simulink model "pet_integration_architecture"  (R2024a)
settings: Solver=FixedStepDiscrete  StartTime=0.0  StopTime=10.0  RelTol=1e-3
undefined symbols (not defined in the file or in its folder): D1, P
undefined symbols (not defined in the file): orig
(part 2 of 3)

== system pet_integration_architecture/Remote Data Server/Local WSL Store ==
  Bus Element In2 : Inport  PortName=win2wsl
  bash Scripts : Subsystem
      settings: PortSchema="{\"entries\":[{\"content\":{\"headerSize\":26,\"margin\":15,\"minimumSpacing\":25,\"sides\":[{\"content\":{},\"type\":\"ConnectorPlacement.EquallySpacedRectSide\",\"uuid\":\"97c1e145-3d4b-49de-9739-71f2af5be190\"},{\"content\":{\"side\":\"RIGHT\"},\"type\":\"ConnectorPlacement.EquallySpacedRectSide\",\"uuid\":\"5a937baa-e46f-4764-8b00-75a1eb9e59b0\"},{\"content\":{\"side\":\"TOP\"},\"type\":\"ConnectorPlacement.EquallySpacedRectSide\",\"uuid\":\"83b91a39-9e34-441d-bccf-4f6b71aa9c87\"}]},\"type\":\"ConnectorPlacement.EquallySpacedConnector\",\"uuid\":\"3f7bec2f-99ca-4d64-b419-ed6b2efa51c2\"}],\"packageUris\":[\"http://schema.mathworks.com/mf0/Connector/R2020b\"],\"version\":\"1.0\"}"
  slurm Jobs : Subsystem
      settings: PortSchema="{\"entries\":[{\"content\":{\"headerSize\":26,\"margin\":15,\"minimumSpacing\":25,\"sides\":[{\"content\":{},\"type\":\"ConnectorPlacement.EquallySpacedRectSide\",\"uuid\":\"97c1e145-3d4b-49de-9739-71f2af5be190\"},{\"content\":{\"side\":\"RIGHT\"},\"type\":\"ConnectorPlacement.EquallySpacedRectSide\",\"uuid\":\"5a937baa-e46f-4764-8b00-75a1eb9e59b0\"},{\"content\":{\"side\":\"TOP\"},\"type\":\"ConnectorPlacement.EquallySpacedRectSide\",\"uuid\":\"83b91a39-9e34-441d-bccf-4f6b71aa9c87\"}]},\"type\":\"ConnectorPlacement.EquallySpacedConnector\",\"uuid\":\"3f7bec2f-99ca-4d64-b419-ed6b2efa51c2\"}],\"packageUris\":[\"http://schema.mathworks.com/mf0/Connector/R2020b\"],\"version\":\"1.0\"}"
  sshConnect : Subsystem
      settings: PortSchema="{\"entries\":[{\"content\":{\"headerSize\":26,\"margin\":15,\"minimumSpacing\":25,\"sides\":[{\"content\":{},\"type\":\"ConnectorPlacement.EquallySpacedRectSide\",\"uuid\":\"97c1e145-3d4b-49de-9739-71f2af5be190\"},{\"content\":{\"side\":\"RIGHT\"},\"type\":\"ConnectorPlacement.EquallySpacedRectSide\",\"uuid\":\"5a937baa-e46f-4764-8b00-75a1eb9e59b0\"},{\"content\":{\"side\":\"TOP\"},\"type\":\"ConnectorPlacement.EquallySpacedRectSide\",\"uuid\":\"83b91a39-9e34-441d-bccf-4f6b71aa9c87\"}]},\"type\":\"ConnectorPlacement.EquallySpacedConnector\",\"uuid\":\"3f7bec2f-99ca-4d64-b419-ed6b2efa51c2\"}],\"packageUris\":[\"http://schema.mathworks.com/mf0/Connector/R2020b\"],\"version\":\"1.0\"}"
  Bus Element Out2 : Outport  AllowServiceAccess=on  PortName=rsync
  Bus Element Out1 : Outport  Port=2  PortName=wsl2win

== system pet_integration_architecture/Remote Data Server/Loris ==

== system pet_integration_architecture/Remote Data Server/Remote Execution Module ==
  Bus Element In1 : Inport  AllowServiceAccess=on  PortName=SSHPort
  In Bus Element1 : Inport  Port=2  PortName=rsync

== system pet_integration_architecture/Remote Data Server/SSH Connection Module ==
  Bus Element In2 : Inport  AllowServiceAccess=on  PortName=rsync
  Bus Element In1 : Inport  Port=2  AllowServiceAccess=on  PortName=SSHPort

== system pet_integration_architecture/Remote Data Server/StormRemote GUI ==

== system pet_integration_architecture/Remote Data Server/WSL Inteface Module ==
  Bus Element In2 : Inport  PortName=wsl2win
  Bus Element In1 : Inport  Port=2  AllowServiceAccess=on  PortName=remote.config
  Bus Element Out1 : Outport  PortName=win2wsl

== system pet_integration_architecture/Remote Data Server/importBIDSDataset ==
  Bus Element In1 : Inport  AllowServiceAccess=on  PortName=local.raw
  Bus Element Out1 : Outport  AllowServiceAccess=on  PortName=Derivatives

== system pet_integration_architecture/brainstorm SQLite Server/Freesurfer Processing Server ==
  Bus Element In1 : Inport  AllowServiceAccess=on  PortName=remote.raw
  PETSurfer : Subsystem
      settings: PortSchema="{\"entries\":[{\"content\":{\"headerSize\":26,\"margin\":15,\"minimumSpacing\":25,\"sides\":[{\"content\":{},\"type\":\"ConnectorPlacement.EquallySpacedRectSide\",\"uuid\":\"d99db108-8c8a-4010-81b2-f142fbf318f5\"},{\"content\":{\"connectorIds\":[\"Out1\"],\"side\":\"RIGHT\"},\"type\":\"ConnectorPlacement.EquallySpacedRectSide\",\"uuid\":\"9190d96c-22e3-4cc9-a507-8f094dc67743\"},{\"content\":{\"side\":\"TOP\"},\"type\":\"ConnectorPlacement.EquallySpacedRectSide\",\"uuid\":\"08b46875-eac1-4edb-b2eb-5598dd517a75\"}]},\"type\":\"ConnectorPlacement.EquallySpacedConnector\",\"uuid\":\"c8d2d02b-cf5a-431f-8876-22d36c8a9b33\"}],\"packageUris\":[\"http://schema.mathworks.com/mf0/Connector/R2020b\"],\"version\":\"1.0\"}"
  recon all : Subsystem
      settings: PortSchema="{\"entries\":[{\"content\":{\"headerSize\":26,\"margin\":15,\"minimumSpacing\":25,\"sides\":[{\"content\":{\"connectorIds\":[\"In1\"]},\"type\":\"ConnectorPlacement.EquallySpacedRectSide\",\"uuid\":\"1ec5f43e-86ec-4420-9dd8-c30b843d5131\"},{\"content\":{\"connectorIds\":[\"Out1\"],\"side\":\"RIGHT\"},\"type\":\"ConnectorPlacement.EquallySpacedRectSide\",\"uuid\":\"372e8174-47dc-4989-909e-f78b7a521fdc\"},{\"content\":{\"side\":\"TOP\"},\"type\":\"ConnectorPlacement.EquallySpacedRectSide\",\"uuid\":\"cc67dfee-4023-44ab-9dd9-de9f078f7d77\"}]},\"type\":\"ConnectorPlacement.EquallySpacedConnector\",\"uuid\":\"fe3e41a6-8f67-44d2-abc6-74b481cf0464\"}],\"packageUris\":[\"http://schema.mathworks.com/mf0/Connector/R2020b\"],\"version\":\"1.0\"}"
  Bus Element Out1 : Outport  PortName=freesurfer derivatives

== system pet_integration_architecture/brainstorm SQLite Server/LORIS Data Ingestor ==

== system pet_integration_architecture/brainstorm SQLite Server/Remote Data Server ==
  Bus Element In1 : Inport  PortName=Derivatives
  " sourceData" : Subsystem
      settings: PortSchema="{\"entries\":[{\"content\":{\"headerSize\":26,\"margin\":15,\"minimumSpacing\":25,\"sides\":[{\"content\":{},\"type\":\"ConnectorPlacement.EquallySpacedRectSide\",\"uuid\":\"a3539b9a-22db-4da3-b271-35b287ced3a1\"},{\"content\":{\"connectorIds\":[\"Out1\"],\"side\":\"RIGHT\"},\"type\":\"ConnectorPlacement.EquallySpacedRectSide\",\"uuid\":\"72d9f298-5062-46d4-b3c5-f2fa85d7a7a6\"},{\"content\":{\"side\":\"TOP\"},\"type\":\"ConnectorPlacement.EquallySpacedRectSide\",\"uuid\":\"050469fd-3881-4b53-a813-94df038aa659\"}]},\"type\":\"ConnectorPlacement.EquallySpacedConnector\",\"uuid\":\"6db04dad-62f3-4987-a6a9-d236db4fe2a3\"}],\"packageUris\":[\"http://schema.mathworks.com/mf0/Connector/R2020b\"],\"version\":\"1.0\"}"
  Home : Subsystem
      settings: PortSchema="{\"entries\":[{\"content\":{\"headerSize\":26,\"margin\":15,\"minimumSpacing\":25,\"sides\":[{\"content\":{\"connectorIds\":[\"Out1\"]},\"type\":\"ConnectorPlacement.EquallySpacedRectSide\",\"uuid\":\"a3539b9a-22db-4da3-b271-35b287ced3a1\"},{\"content\":{\"side\":\"RIGHT\"},\"type\":\"ConnectorPlacement.EquallySpacedRectSide\",\"uuid\":\"72d9f298-5062-46d4-b3c5-f2fa85d7a7a6\"},{\"content\":{\"side\":\"TOP\"},\"type\":\"ConnectorPlacement.EquallySpacedRectSide\",\"uuid\":\"050469fd-3881-4b53-a813-94df038aa659\"}]},\"type\":\"ConnectorPlacement.EquallySpacedConnector\",\"uuid\":\"6db04dad-62f3-4987-a6a9-d236db4fe2a3\"}],\"packageUris\":[\"http://schema.mathworks.com/mf0/Connector/R2020b\"],\"version\":\"1.0\"}"
  derivativesData : Subsystem
      settings: PortSchema="{\"entries\":[{\"content\":{\"headerSize\":26,\"margin\":15,\"minimumSpacing\":25,\"sides\":[{\"content\":{},\"type\":\"ConnectorPlacement.EquallySpacedRectSide\",\"uuid\":\"a3539b9a-22db-4da3-b271-35b287ced3a1\"},{\"content\":{\"side\":\"RIGHT\"},\"type\":\"ConnectorPlacement.EquallySpacedRectSide\",\"uuid\":\"72d9f298-5062-46d4-b3c5-f2fa85d7a7a6\"},{\"content\":{\"side\":\"TOP\"},\"type\":\"ConnectorPlacement.EquallySpacedRectSide\",\"uuid\":\"050469fd-3881-4b53-a813-94df038aa659\"}]},\"type\":\"ConnectorPlacement.EquallySpacedConnector\",\"uuid\":\"6db04dad-62f3-4987-a6a9-d236db4fe2a3\"}],\"packageUris\":[\"http://schema.mathworks.com/mf0/Connector/R2020b\"],\"version\":\"1.0\"}"
  Bus Element Out4 : Outport  AllowServiceAccess=on  PortName=sourceCode  Element=github
  Bus Element Out3 : Outport  Port=2  AllowServiceAccess=on  PortName=SSHPort
  Bus Element Out1 : Outport  Port=3  AllowServiceAccess=on  PortName=remote.raw
  Bus Element Out2 : Outport  Port=4  AllowServiceAccess=on  PortName=remote.derivatives
  wires:
  " sourceData"/1(remote) -> Bus Element Out1/1, Bus Element Out2/1
  Home/1(sourceCode) -> Bus Element Out4/1

== system pet_integration_architecture/brainstorm SQLite Server/create Virtual Environment ==

== system pet_integration_architecture/brainstorm SQLite Server/gitClone Brainstorm ==
  Bus Element In1 : Inport  AllowServiceAccess=on  PortName=sourceCode

== system pet_integration_architecture/brainstorm SQLite Server/jobScheduler ==

== system pet_integration_architecture/brainstorm SQLite Server/loadPython ==

== system pet_integration_architecture/brainstorm SQLite Server/processingSoftware ==

== system pet_integration_architecture/brainstorm core/bst_get ==

== system pet_integration_architecture/brainstorm core/bst_set ==

== system pet_integration_architecture/brainstorm database/Brainstorm Home Dir ==

== system pet_integration_architecture/brainstorm database/Brainstorm User Data  ==

== system pet_integration_architecture/brainstorm database/Brainstorm data server ==
  note: data directory
  note: anat directory
  note: /anat/subName/subject/
  note: /data/subName/@raw/
  Bus Element In1 : Inport  PortName=@db
  channel_ : Subsystem
      settings: PortSchema="{\"entries\":[{\"content\":{\"headerSize\":26,\"margin\":15,\"minimumSpacing\":25,\"sides\":[{\"content\":{\"connectorIds\":[\"In1\"]},\"type\":\"ConnectorPlacement.EquallySpacedRectSide\",\"uuid\":\"e452b68a-48a0-46a4-9e6b-6a7ab63d76ba\"},{\"content\":{\"side\":\"RIGHT\"},\"type\":\"ConnectorPlacement.EquallySpacedRectSide\",\"uuid\":\"bfc23a96-7562-4108-a377-c6d682106293\"},{\"content\":{\"side\":\"TOP\"},\"type\":\"ConnectorPlacement.EquallySpacedRectSide\",\"uuid\":\"898805eb-9365-4e37-9830-3cdbb7191da7\"}]},\"type\":\"ConnectorPlacement.EquallySpacedConnector\",\"uuid\":\"9a83eb3e-c81f-4df4-a7ca-e8a116b52f55\"}],\"packageUris\":[\"http://schema.mathworks.com/mf0/Connector/R2020b\"],\"version\":\"1.0\"}"
  channel_1 : Subsystem
      settings: PortSchema="{\"entries\":[{\"content\":{\"headerSize\":26,\"margin\":15,\"minimumSpacing\":25,\"sides\":[{\"content\":{\"connectorIds\":[\"In1\"]},\"type\":\"ConnectorPlacement.EquallySpacedRectSide\",\"uuid\":\"e452b68a-48a0-46a4-9e6b-6a7ab63d76ba\"},{\"content\":{\"side\":\"RIGHT\"},\"type\":\"ConnectorPlacement.EquallySpacedRectSide\",\"uuid\":\"bfc23a96-7562-4108-a377-c6d682106293\"},{\"content\":{\"side\":\"TOP\"},\"type\":\"ConnectorPlacement.EquallySpacedRectSide\",\"uuid\":\"898805eb-9365-4e37-9830-3cdbb7191da7\"}]},\"type\":\"ConnectorPlacement.EquallySpacedConnector\",\"uuid\":\"9a83eb3e-c81f-4df4-a7ca-e8a116b52f55\"}],\"packageUris\":[\"http://schema.mathworks.com/mf0/Connector/R2020b\"],\"version\":\"1.0\"}"
  data_ : Subsystem
      settings: PortSchema="{\"entries\":[{\"content\":{\"headerSize\":26,\"margin\":15,\"minimumSpacing\":25,\"sides\":[{\"content\":{\"connectorIds\":[\"In1\"]},\"type\":\"ConnectorPlacement.EquallySpacedRectSide\",\"uuid\":\"e452b68a-48a0-46a4-9e6b-6a7ab63d76ba\"},{\"content\":{\"side\":\"RIGHT\"},\"type\":\"ConnectorPlacement.EquallySpacedRectSide\",\"uuid\":\"bfc23a96-7562-4108-a377-c6d682106293\"},{\"content\":{\"side\":\"TOP\"},\"type\":\"ConnectorPlacement.EquallySpacedRectSide\",\"uuid\":\"898805eb-9365-4e37-9830-3cdbb7191da7\"}]},\"type\":\"ConnectorPlacement.EquallySpacedConnector\",\"uuid\":\"9a83eb3e-c81f-4df4-a7ca-e8a116b52f55\"}],\"packageUris\":[\"http://schema.mathworks.com/mf0/Connector/R2020b\"],\"version\":\"1.0\"}"
  pet_ : Subsystem
      settings: PortSchema="{\"entries\":[{\"content\":{\"headerSize\":26,\"margin\":15,\"minimumSpacing\":25,\"sides\":[{\"content\":{\"connectorIds\":[\"In1\",\"In2\",\"In3\"]},\"type\":\"ConnectorPlacement.EquallySpacedRectSide\",\"uuid\":\"e452b68a-48a0-46a4-9e6b-6a7ab63d76ba\"},{\"content\":{\"side\":\"RIGHT\"},\"type\":\"ConnectorPlacement.EquallySpacedRectSide\",\"uuid\":\"bfc23a96-7562-4108-a377-c6d682106293\"},{\"content\":{\"side\":\"TOP\"},\"type\":\"ConnectorPlacement.EquallySpacedRectSide\",\"uuid\":\"898805eb-9365-4e37-9830-3cdbb7191da7\"},{\"content\":{\"side\":\"BOTTOM\"},\"type\":\"ConnectorPlacement.EquallySpacedRectSide\",\"uuid\":\"351f7cf8-f356-44ed-a891-6a23a007c224\"}]},\"type\":\"ConnectorPlacement.EquallySpacedConnector\",\"uuid\":\"9a83eb3e-c81f-4df4-a7ca-e8a116b52f55\"}],\"packageUris\":[\"http://schema.mathworks.com/mf0/Connector/R2020b\"],\"version\":\"1.0\"}"
  subjectimage_ : Subsystem
      settings: PortSchema="{\"entries\":[{\"content\":{\"headerSize\":26,\"margin\":15,\"minimumSpacing\":25,\"sides\":[{\"content\":{\"connectorIds\":[\"In1\"]},\"type\":\"ConnectorPlacement.EquallySpacedRectSide\",\"uuid\":\"e452b68a-48a0-46a4-9e6b-6a7ab63d76ba\"},{\"content\":{\"side\":\"RIGHT\"},\"type\":\"ConnectorPlacement.EquallySpacedRectSide\",\"uuid\":\"bfc23a96-7562-4108-a377-c6d682106293\"},{\"content\":{\"side\":\"TOP\"},\"type\":\"ConnectorPlacement.EquallySpacedRectSide\",\"uuid\":\"898805eb-9365-4e37-9830-3cdbb7191da7\"}]},\"type\":\"ConnectorPlacement.EquallySpacedConnector\",\"uuid\":\"9a83eb3e-c81f-4df4-a7ca-e8a116b52f55\"}],\"packageUris\":[\"http://schema.mathworks.com/mf0/Connector/R2020b\"],\"version\":\"1.0\"}"
  tess_ : Subsystem
      settings: PortSchema="{\"entries\":[{\"content\":{\"headerSize\":26,\"margin\":15,\"minimumSpacing\":25,\"sides\":[{\"content\":{\"connectorIds\":[\"In1\"]},\"type\":\"ConnectorPlacement.EquallySpacedRectSide\",\"uuid\":\"e452b68a-48a0-46a4-9e6b-6a7ab63d76ba\"},{\"content\":{\"side\":\"RIGHT\"},\"type\":\"ConnectorPlacement.EquallySpacedRectSide\",\"uuid\":\"bfc23a96-7562-4108-a377-c6d682106293\"},{\"content\":{\"side\":\"TOP\"},\"type\":\"ConnectorPlacement.EquallySpacedRectSide\",\"uuid\":\"898805eb-9365-4e37-9830-3cdbb7191da7\"}]},\"type\":\"ConnectorPlacement.EquallySpacedConnector\",\"uuid\":\"9a83eb3e-c81f-4df4-a7ca-e8a116b52f55\"}],\"packageUris\":[\"http://schema.mathworks.com/mf0/Connector/R2020b\"],\"version\":\"1.0\"}"
  Bus Element Out1 : Outport  PortName=in_(@varargin)
  wires:
  ? -> pet_/1(FileName)
  ? -> pet_/2(Tracer)
  ? -> pet_/3(nFrames)

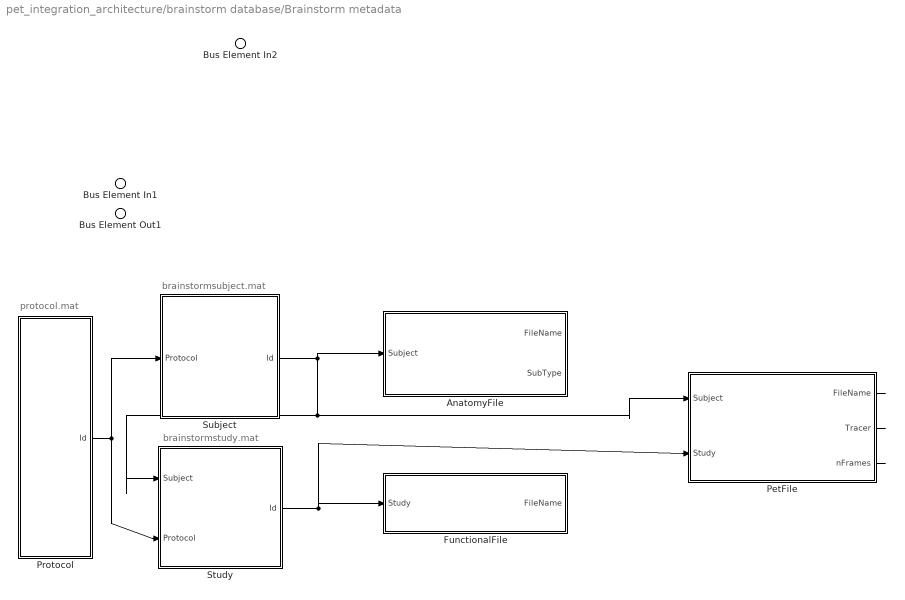
== system pet_integration_architecture/brainstorm database/Brainstorm metadata  ==
  note: brainstormsubject.mat
  note: protocol.mat
  note: brainstormstudy.mat
  Bus Element In2 : Inport  PortName=bst_set(@db)
  Bus Element In1 : Inport  Port=2  AllowServiceAccess=on  PortName=TCP1433Port
  AnatomyFile : Subsystem
      settings: PortSchema="{\"entries\":[{\"content\":{\"headerSize\":26,\"margin\":15,\"minimumSpacing\":25,\"sides\":[{\"content\":{\"connectorIds\":[\"In1\"]},\"type\":\"ConnectorPlacement.EquallySpacedRectSide\",\"uuid\":\"e452b68a-48a0-46a4-9e6b-6a7ab63d76ba\"},{\"content\":{\"connectorIds\":[\"Out1\",\"Out2\"],\"side\":\"RIGHT\"},\"type\":\"ConnectorPlacement.EquallySpacedRectSide\",\"uuid\":\"bfc23a96-7562-4108-a377-c6d682106293\"},{\"content\":{\"side\":\"TOP\"},\"type\":\"ConnectorPlacement.EquallySpacedRectSide\",\"uuid\":\"898805eb-9365-4e37-9830-3cdbb7191da7\"}]},\"type\":\"ConnectorPlacement.EquallySpacedConnector\",\"uuid\":\"9a83eb3e-c81f-4df4-a7ca-e8a116b52f55\"}],\"packageUris\":[\"http://schema.mathworks.com/mf0/Connector/R2020b\"],\"version\":\"1.0\"}"
  FunctionalFile : Subsystem
      settings: PortSchema="{\"entries\":[{\"content\":{\"headerSize\":26,\"margin\":15,\"minimumSpacing\":25,\"sides\":[{\"content\":{\"connectorIds\":[\"In1\"]},\"type\":\"ConnectorPlacement.EquallySpacedRectSide\",\"uuid\":\"d9face5b-155e-4e83-95c0-d581b737b6e3\"},{\"content\":{\"connectorIds\":[\"Out1\"],\"side\":\"RIGHT\"},\"type\":\"ConnectorPlacement.EquallySpacedRectSide\",\"uuid\":\"f965be1f-1639-4140-b9ea-f5e9efbe4150\"},{\"content\":{\"side\":\"TOP\"},\"type\":\"ConnectorPlacement.EquallySpacedRectSide\",\"uuid\":\"7c9c4b2b-011c-4482-afab-b6e67025a5e2\"}]},\"type\":\"ConnectorPlacement.EquallySpacedConnector\",\"uuid\":\"ec963004-117d-4f22-bb00-71f35201e6e2\"}],\"packageUris\":[\"http://schema.mathworks.com/mf0/Connector/R2020b\"],\"version\":\"1.0\"}"
  PetFile : Subsystem
      settings: AttributesFormatString=%<RequirementInfo>  PortSchema="{\"entries\":[{\"content\":{\"headerSize\":26,\"margin\":15,\"minimumSpacing\":25,\"sides\":[{\"content\":{\"connectorIds\":[\"In2\",\"In1\"]},\"type\":\"ConnectorPlacement.EquallySpacedRectSide\",\"uuid\":\"d9face5b-155e-4e83-95c0-d581b737b6e3\"},{\"content\":{\"connectorIds\":[\"Out1\",\"Out2\",\"Out3\"],\"side\":\"RIGHT\"},\"type\":\"ConnectorPlacement.EquallySpacedRectSide\",\"uuid\":\"f965be1f-1639-4140-b9ea-f5e9efbe4150\"},{\"content\":{\"side\":\"TOP\"},\"type\":\"ConnectorPlacement.EquallySpacedRectSide\",\"uuid\":\"7c9c4b2b-011c-4482-afab-b6e67025a5e2\"}]},\"type\":\"ConnectorPlacement.EquallySpacedConnector\",\"uuid\":\"ec963004-117d-4f22-bb00-71f35201e6e2\"}],\"packageUris\":[\"http://schema.mathworks.com/mf0/Connector/R2020b\"],\"version\":\"1.0\"}"
  Protocol : Subsystem
      settings: PortSchema="{\"entries\":[{\"content\":{\"headerSize\":26,\"margin\":15,\"minimumSpacing\":25,\"sides\":[{\"content\":{},\"type\":\"ConnectorPlacement.EquallySpacedRectSide\",\"uuid\":\"e452b68a-48a0-46a4-9e6b-6a7ab63d76ba\"},{\"content\":{\"connectorIds\":[\"Out1\"],\"side\":\"RIGHT\"},\"type\":\"ConnectorPlacement.EquallySpacedRectSide\",\"uuid\":\"bfc23a96-7562-4108-a377-c6d682106293\"},{\"content\":{\"side\":\"TOP\"},\"type\":\"ConnectorPlacement.EquallySpacedRectSide\",\"uuid\":\"898805eb-9365-4e37-9830-3cdbb7191da7\"}]},\"type\":\"ConnectorPlacement.EquallySpacedConnector\",\"uuid\":\"9a83eb3e-c81f-4df4-a7ca-e8a116b52f55\"}],\"packageUris\":[\"http://schema.mathworks.com/mf0/Connector/R2020b\"],\"version\":\"1.0\"}"
  Study : Subsystem
      settings: PortSchema="{\"entries\":[{\"content\":{\"headerSize\":26,\"margin\":15,\"minimumSpacing\":25,\"sides\":[{\"content\":{\"connectorIds\":[\"In2\",\"In1\"]},\"type\":\"ConnectorPlacement.EquallySpacedRectSide\",\"uuid\":\"d9face5b-155e-4e83-95c0-d581b737b6e3\"},{\"content\":{\"connectorIds\":[\"Out1\"],\"side\":\"RIGHT\"},\"type\":\"ConnectorPlacement.EquallySpacedRectSide\",\"uuid\":\"f965be1f-1639-4140-b9ea-f5e9efbe4150\"},{\"content\":{\"side\":\"TOP\"},\"type\":\"ConnectorPlacement.EquallySpacedRectSide\",\"uuid\":\"7c9c4b2b-011c-4482-afab-b6e67025a5e2\"}]},\"type\":\"ConnectorPlacement.EquallySpacedConnector\",\"uuid\":\"ec963004-117d-4f22-bb00-71f35201e6e2\"}],\"packageUris\":[\"http://schema.mathworks.com/mf0/Connector/R2020b\"],\"version\":\"1.0\"}"
  Subject : Subsystem
      settings: PortSchema="{\"entries\":[{\"content\":{\"headerSize\":26,\"margin\":15,\"minimumSpacing\":25,\"sides\":[{\"content\":{\"connectorIds\":[\"In1\"]},\"type\":\"ConnectorPlacement.EquallySpacedRectSide\",\"uuid\":\"d9face5b-155e-4e83-95c0-d581b737b6e3\"},{\"content\":{\"connectorIds\":[\"Out1\"],\"side\":\"RIGHT\"},\"type\":\"ConnectorPlacement.EquallySpacedRectSide\",\"uuid\":\"f965be1f-1639-4140-b9ea-f5e9efbe4150\"},{\"content\":{\"side\":\"TOP\"},\"type\":\"ConnectorPlacement.EquallySpacedRectSide\",\"uuid\":\"7c9c4b2b-011c-4482-afab-b6e67025a5e2\"}]},\"type\":\"ConnectorPlacement.EquallySpacedConnector\",\"uuid\":\"ec963004-117d-4f22-bb00-71f35201e6e2\"}],\"packageUris\":[\"http://schema.mathworks.com/mf0/Connector/R2020b\"],\"version\":\"1.0\"}"
  Bus Element Out1 : Outport  PortName=bst_get(@db)
  wires:
  Study/1(Id) -> FunctionalFile/1(Study), PetFile/1(Study)
  Protocol/1(Id) -> Study/1(Protocol), Subject/1(Protocol)
  Subject/1(Id) -> Study/2(Subject), PetFile/2(Subject), AnatomyFile/1(Subject)
  PetFile/1(FileName) -> ?
  PetFile/2(Tracer) -> ?
  PetFile/3(nFrames) -> ?

== system pet_integration_architecture/brainstorm gui/gui_component ('Import PET') ==
  Bus Element Out1 : Outport  PortName=gui_callback

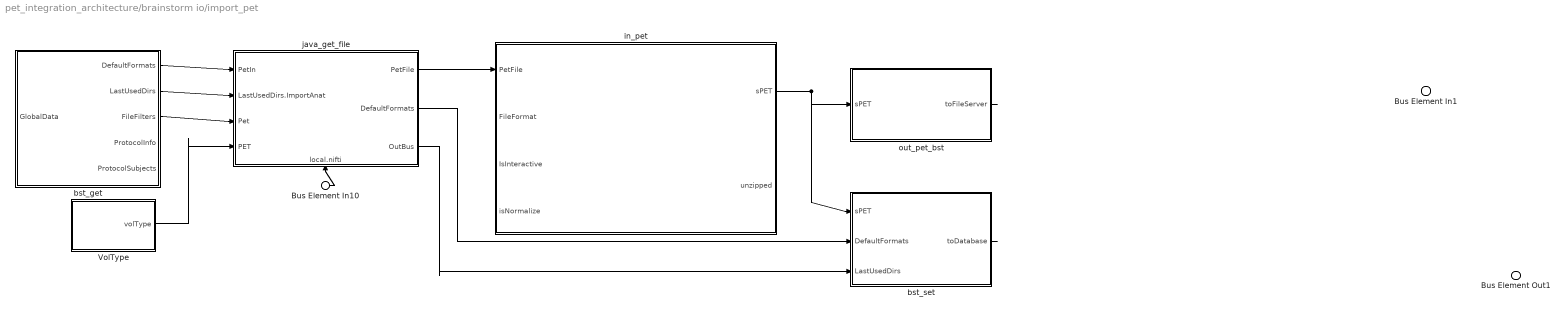
== system pet_integration_architecture/brainstorm io/import_pet ==
  Bus Element In1 : Inport  PortName=impet_in
  Bus Element In10 : Inport  Port=2  AllowServiceAccess=on  PortName=local.nifti
  VolType : Subsystem
      settings: PortSchema="{\"entries\":[{\"content\":{\"headerSize\":26,\"margin\":15,\"minimumSpacing\":25,\"sides\":[{\"content\":{},\"type\":\"ConnectorPlacement.EquallySpacedRectSide\",\"uuid\":\"9dc41937-0423-4f0d-95de-6a11876dea92\"},{\"content\":{\"connectorIds\":[\"Out1\"],\"side\":\"RIGHT\"},\"type\":\"ConnectorPlacement.EquallySpacedRectSide\",\"uuid\":\"a760f902-bb88-44c6-9e15-f93a06bbb22c\"},{\"content\":{\"side\":\"TOP\"},\"type\":\"ConnectorPlacement.EquallySpacedRectSide\",\"uuid\":\"a141426c-a194-4d5c-ba1a-f6f4f49c40a6\"}]},\"type\":\"ConnectorPlacement.EquallySpacedConnector\",\"uuid\":\"ec924d27-401c-47e0-a07a-aece678b254f\"}],\"packageUris\":[\"http://schema.mathworks.com/mf0/Connector/R2020b\"],\"version\":\"1.0\"}"
  bst_get : Subsystem
      settings: PortSchema="{\"entries\":[{\"content\":{\"headerSize\":26,\"margin\":15,\"minimumSpacing\":25,\"sides\":[{\"content\":{\"connectorIds\":[\"In1\"]},\"type\":\"ConnectorPlacement.EquallySpacedRectSide\",\"uuid\":\"e452b68a-48a0-46a4-9e6b-6a7ab63d76ba\"},{\"content\":{\"connectorIds\":[\"Out1\",\"Out2\",\"Out3\",\"Out4\",\"Out5\"],\"side\":\"RIGHT\"},\"type\":\"ConnectorPlacement.EquallySpacedRectSide\",\"uuid\":\"bfc23a96-7562-4108-a377-c6d682106293\"},{\"content\":{\"side\":\"TOP\"},\"type\":\"ConnectorPlacement.EquallySpacedRectSide\",\"uuid\":\"898805eb-9365-4e37-9830-3cdbb7191da7\"}]},\"type\":\"ConnectorPlacement.EquallySpacedConnector\",\"uuid\":\"9a83eb3e-c81f-4df4-a7ca-e8a116b52f55\"}],\"packageUris\":[\"http://schema.mathworks.com/mf0/Connector/R2020b\"],\"version\":\"1.0\"}"
  bst_set : Subsystem
      settings: PortSchema="{\"entries\":[{\"content\":{\"headerSize\":26,\"margin\":15,\"minimumSpacing\":25,\"sides\":[{\"content\":{\"connectorIds\":[\"In1\",\"In2\",\"In3\"]},\"type\":\"ConnectorPlacement.EquallySpacedRectSide\",\"uuid\":\"e452b68a-48a0-46a4-9e6b-6a7ab63d76ba\"},{\"content\":{\"connectorIds\":[\"Out1\"],\"side\":\"RIGHT\"},\"type\":\"ConnectorPlacement.EquallySpacedRectSide\",\"uuid\":\"bfc23a96-7562-4108-a377-c6d682106293\"},{\"content\":{\"side\":\"TOP\"},\"type\":\"ConnectorPlacement.EquallySpacedRectSide\",\"uuid\":\"898805eb-9365-4e37-9830-3cdbb7191da7\"}]},\"type\":\"ConnectorPlacement.EquallySpacedConnector\",\"uuid\":\"9a83eb3e-c81f-4df4-a7ca-e8a116b52f55\"}],\"packageUris\":[\"http://schema.mathworks.com/mf0/Connector/R2020b\"],\"version\":\"1.0\"}"
  in_pet : Subsystem
      settings: PortSchema="{\"entries\":[{\"content\":{\"headerSize\":26,\"margin\":15,\"minimumSpacing\":25,\"sides\":[{\"content\":{\"connectorIds\":[\"In4\",\"In1\",\"In2\",\"In3\"]},\"type\":\"ConnectorPlacement.EquallySpacedRectSide\",\"uuid\":\"e452b68a-48a0-46a4-9e6b-6a7ab63d76ba\"},{\"content\":{\"connectorIds\":[\"Out1\",\"Out2\"],\"side\":\"RIGHT\"},\"type\":\"ConnectorPlacement.EquallySpacedRectSide\",\"uuid\":\"bfc23a96-7562-4108-a377-c6d682106293\"},{\"content\":{\"side\":\"TOP\"},\"type\":\"ConnectorPlacement.EquallySpacedRectSide\",\"uuid\":\"898805eb-9365-4e37-9830-3cdbb7191da7\"}]},\"type\":\"ConnectorPlacement.EquallySpacedConnector\",\"uuid\":\"9a83eb3e-c81f-4df4-a7ca-e8a116b52f55\"}],\"packageUris\":[\"http://schema.mathworks.com/mf0/Connector/R2020b\"],\"version\":\"1.0\"}"
  java_get_file : Subsystem
      settings: PortSchema="{\"entries\":[{\"content\":{\"headerSize\":26,\"margin\":15,\"minimumSpacing\":25,\"sides\":[{\"content\":{\"connectorIds\":[\"In2\",\"In1\",\"In3\",\"In4\"]},\"type\":\"ConnectorPlacement.EquallySpacedRectSide\",\"uuid\":\"d9face5b-155e-4e83-95c0-d581b737b6e3\"},{\"content\":{\"connectorIds\":[\"Out1\",\"Out2\",\"Out3\"],\"side\":\"RIGHT\"},\"type\":\"ConnectorPlacement.EquallySpacedRectSide\",\"uuid\":\"f965be1f-1639-4140-b9ea-f5e9efbe4150\"},{\"content\":{\"side\":\"TOP\"},\"type\":\"ConnectorPlacement.EquallySpacedRectSide\",\"uuid\":\"7c9c4b2b-011c-4482-afab-b6e67025a5e2\"},{\"content\":{\"connectorIds\":[\"In5\"],\"side\":\"BOTTOM\"},\"type\":\"ConnectorPlacement.EquallySpacedRectSide\",\"uuid\":\"d045f323-f36b-4304-ab53-40ed85860a49\"}]},\"type\":\"ConnectorPlacement.EquallySpacedConnector\",\"uuid\":\"ec963004-117d-4f22-bb00-71f35201e6e2\"}],\"packageUris\":[\"http://schema.mathworks.com/mf0/Connector/R2020b\"],\"version\":\"1.0\"}"
  out_pet_bst : Subsystem
      settings: PortSchema="{\"entries\":[{\"content\":{\"headerSize\":26,\"margin\":15,\"minimumSpacing\":25,\"sides\":[{\"content\":{\"connectorIds\":[\"In1\"]},\"type\":\"ConnectorPlacement.EquallySpacedRectSide\",\"uuid\":\"b493315f-c6c8-42ab-8e4d-b8fe240af9dd\"},{\"content\":{\"connectorIds\":[\"Out1\"],\"side\":\"RIGHT\"},\"type\":\"ConnectorPlacement.EquallySpacedRectSide\",\"uuid\":\"94c0e42b-c474-4070-8a16-a26ac22942e6\"},{\"content\":{\"side\":\"TOP\"},\"type\":\"ConnectorPlacement.EquallySpacedRectSide\",\"uuid\":\"f9bc43e9-5c3a-451c-b434-9225c48927cc\"}]},\"type\":\"ConnectorPlacement.EquallySpacedConnector\",\"uuid\":\"067458af-ee7c-44e6-8802-98d558b25815\"}],\"packageUris\":[\"http://schema.mathworks.com/mf0/Connector/R2020b\"],\"version\":\"1.0\"}"
  Bus Element Out1 : Outport  PortName=impet_out
  wires:
  bst_get/3(FileFilters) -> java_get_file/3(Pet)
  bst_get/2(LastUsedDirs) -> java_get_file/1(LastUsedDirs.ImportAnat)
  bst_get/1(DefaultFormats) -> java_get_file/2(PetIn)
  Bus Element In10/1 -> java_get_file/5(local.nifti)
  java_get_file/1(PetFile) -> in_pet/4(PetFile)
  java_get_file/2(DefaultFormats) -> bst_set/2(DefaultFormats)
  java_get_file/3(OutBus) -> bst_set/3(LastUsedDirs)
  VolType/1(volType) -> java_get_file/4(PET)
  in_pet/1(sPET) -> bst_set/1(sPET), out_pet_bst/1(sPET)
  out_pet_bst/1(toFileServer) -> ?
  bst_set/1(toDatabase) -> ?

== system pet_integration_architecture/brainstorm tools/Anatomy ==
  Bus Element Out2 : Outport  AllowServiceAccess=on  PortName=Surface Recon
  Bus Element Out1 : Outport  Port=2  AllowServiceAccess=on  PortName=BstMriFile

== system pet_integration_architecture/brainstorm tools/bst_colormaps ==

== system pet_integration_architecture/brainstorm tools/bst_get ==
  Bus Element In2 : Inport  PortName=bst_get(@db)
  Out Bus Element1 : Outport  PortName=io

== system pet_integration_architecture/brainstorm tools/bst_memory ==

== system pet_integration_architecture/brainstorm tools/bst_set ==
  Bus Element In1 : Inport  PortName=io
  Out Bus Element1 : Outport  PortName=bst_set(@db)

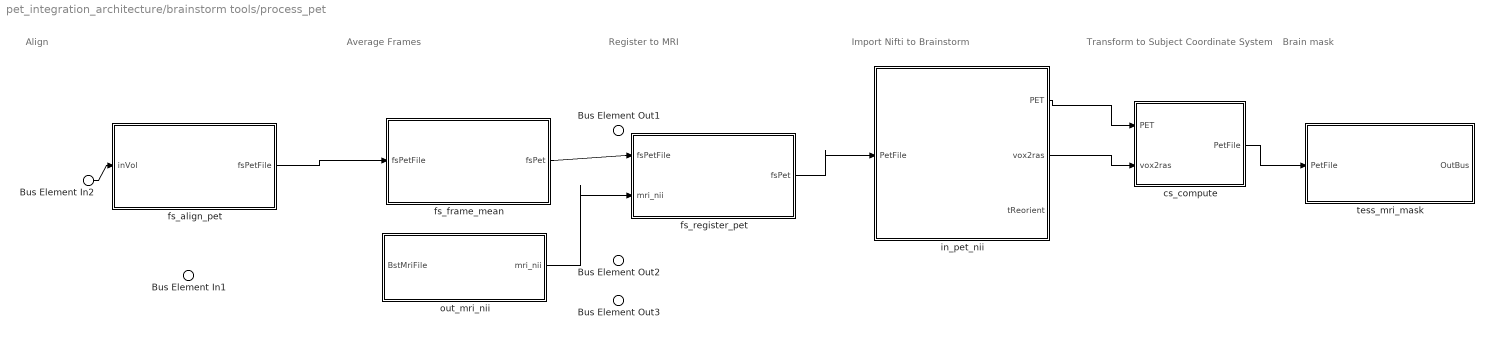
== system pet_integration_architecture/brainstorm tools/process_pet ==
  note: Average Frames
  note: Import Nifti to Brainstorm
  note: Brain mask
  note: Register to MRI
  note: Align
  note: Transform to
      | Subject Coordinate System
  Bus Element In2 : Inport  PortName=PetFile
  Bus Element In1 : Inport  Port=2  AllowServiceAccess=on  PortName=BstMriFile
  cs_compute : Subsystem
      settings: PortSchema="{\"entries\":[{\"content\":{\"headerSize\":26,\"margin\":15,\"minimumSpacing\":25,\"sides\":[{\"content\":{\"connectorIds\":[\"In1\",\"In2\"]},\"type\":\"ConnectorPlacement.EquallySpacedRectSide\",\"uuid\":\"d9face5b-155e-4e83-95c0-d581b737b6e3\"},{\"content\":{\"connectorIds\":[\"Out1\"],\"side\":\"RIGHT\"},\"type\":\"ConnectorPlacement.EquallySpacedRectSide\",\"uuid\":\"f965be1f-1639-4140-b9ea-f5e9efbe4150\"},{\"content\":{\"side\":\"TOP\"},\"type\":\"ConnectorPlacement.EquallySpacedRectSide\",\"uuid\":\"7c9c4b2b-011c-4482-afab-b6e67025a5e2\"}]},\"type\":\"ConnectorPlacement.EquallySpacedConnector\",\"uuid\":\"ec963004-117d-4f22-bb00-71f35201e6e2\"}],\"packageUris\":[\"http://schema.mathworks.com/mf0/Connector/R2020b\"],\"version\":\"1.0\"}"
  fs_align_pet : Subsystem
      settings: PortSchema="{\"entries\":[{\"content\":{\"headerSize\":26,\"margin\":15,\"minimumSpacing\":25,\"sides\":[{\"content\":{\"connectorIds\":[\"In1\"]},\"type\":\"ConnectorPlacement.EquallySpacedRectSide\",\"uuid\":\"d9face5b-155e-4e83-95c0-d581b737b6e3\"},{\"content\":{\"connectorIds\":[\"Out1\"],\"side\":\"RIGHT\"},\"type\":\"ConnectorPlacement.EquallySpacedRectSide\",\"uuid\":\"f965be1f-1639-4140-b9ea-f5e9efbe4150\"},{\"content\":{\"side\":\"TOP\"},\"type\":\"ConnectorPlacement.EquallySpacedRectSide\",\"uuid\":\"7c9c4b2b-011c-4482-afab-b6e67025a5e2\"}]},\"type\":\"ConnectorPlacement.EquallySpacedConnector\",\"uuid\":\"ec963004-117d-4f22-bb00-71f35201e6e2\"}],\"packageUris\":[\"http://schema.mathworks.com/mf0/Connector/R2020b\"],\"version\":\"1.0\"}"
  fs_frame_mean : Subsystem
      settings: PortSchema="{\"entries\":[{\"content\":{\"headerSize\":26,\"margin\":15,\"minimumSpacing\":25,\"sides\":[{\"content\":{\"connectorIds\":[\"In1\"]},\"type\":\"ConnectorPlacement.EquallySpacedRectSide\",\"uuid\":\"d9face5b-155e-4e83-95c0-d581b737b6e3\"},{\"content\":{\"connectorIds\":[\"Out1\"],\"side\":\"RIGHT\"},\"type\":\"ConnectorPlacement.EquallySpacedRectSide\",\"uuid\":\"f965be1f-1639-4140-b9ea-f5e9efbe4150\"},{\"content\":{\"side\":\"TOP\"},\"type\":\"ConnectorPlacement.EquallySpacedRectSide\",\"uuid\":\"7c9c4b2b-011c-4482-afab-b6e67025a5e2\"}]},\"type\":\"ConnectorPlacement.EquallySpacedConnector\",\"uuid\":\"ec963004-117d-4f22-bb00-71f35201e6e2\"}],\"packageUris\":[\"http://schema.mathworks.com/mf0/Connector/R2020b\"],\"version\":\"1.0\"}"
  fs_register_pet : Subsystem
      settings: PortSchema="{\"entries\":[{\"content\":{\"headerSize\":26,\"margin\":15,\"minimumSpacing\":25,\"sides\":[{\"content\":{\"connectorIds\":[\"In1\",\"In2\"]},\"type\":\"ConnectorPlacement.EquallySpacedRectSide\",\"uuid\":\"d9face5b-155e-4e83-95c0-d581b737b6e3\"},{\"content\":{\"connectorIds\":[\"Out1\"],\"side\":\"RIGHT\"},\"type\":\"ConnectorPlacement.EquallySpacedRectSide\",\"uuid\":\"f965be1f-1639-4140-b9ea-f5e9efbe4150\"},{\"content\":{\"side\":\"TOP\"},\"type\":\"ConnectorPlacement.EquallySpacedRectSide\",\"uuid\":\"7c9c4b2b-011c-4482-afab-b6e67025a5e2\"}]},\"type\":\"ConnectorPlacement.EquallySpacedConnector\",\"uuid\":\"ec963004-117d-4f22-bb00-71f35201e6e2\"}],\"packageUris\":[\"http://schema.mathworks.com/mf0/Connector/R2020b\"],\"version\":\"1.0\"}"
  in_pet_nii : Subsystem
      settings: PortSchema="{\"entries\":[{\"content\":{\"headerSize\":26,\"margin\":15,\"minimumSpacing\":25,\"sides\":[{\"content\":{\"connectorIds\":[\"In1\"]},\"type\":\"ConnectorPlacement.EquallySpacedRectSide\",\"uuid\":\"d9face5b-155e-4e83-95c0-d581b737b6e3\"},{\"content\":{\"connectorIds\":[\"Out1\",\"Out2\",\"Out3\"],\"side\":\"RIGHT\"},\"type\":\"ConnectorPlacement.EquallySpacedRectSide\",\"uuid\":\"f965be1f-1639-4140-b9ea-f5e9efbe4150\"},{\"content\":{\"side\":\"TOP\"},\"type\":\"ConnectorPlacement.EquallySpacedRectSide\",\"uuid\":\"7c9c4b2b-011c-4482-afab-b6e67025a5e2\"}]},\"type\":\"ConnectorPlacement.EquallySpacedConnector\",\"uuid\":\"ec963004-117d-4f22-bb00-71f35201e6e2\"}],\"packageUris\":[\"http://schema.mathworks.com/mf0/Connector/R2020b\"],\"version\":\"1.0\"}"
  out_mri_nii : Subsystem
      settings: PortSchema="{\"entries\":[{\"content\":{\"headerSize\":26,\"margin\":15,\"minimumSpacing\":25,\"sides\":[{\"content\":{\"connectorIds\":[\"In1\"]},\"type\":\"ConnectorPlacement.EquallySpacedRectSide\",\"uuid\":\"d9face5b-155e-4e83-95c0-d581b737b6e3\"},{\"content\":{\"connectorIds\":[\"Out1\"],\"side\":\"RIGHT\"},\"type\":\"ConnectorPlacement.EquallySpacedRectSide\",\"uuid\":\"f965be1f-1639-4140-b9ea-f5e9efbe4150\"},{\"content\":{\"side\":\"TOP\"},\"type\":\"ConnectorPlacement.EquallySpacedRectSide\",\"uuid\":\"7c9c4b2b-011c-4482-afab-b6e67025a5e2\"}]},\"type\":\"ConnectorPlacement.EquallySpacedConnector\",\"uuid\":\"ec963004-117d-4f22-bb00-71f35201e6e2\"}],\"packageUris\":[\"http://schema.mathworks.com/mf0/Connector/R2020b\"],\"version\":\"1.0\"}"
  tess_mri_mask : Subsystem
      settings: PortSchema="{\"entries\":[{\"content\":{\"headerSize\":26,\"margin\":15,\"minimumSpacing\":25,\"sides\":[{\"content\":{\"connectorIds\":[\"In1\"]},\"type\":\"ConnectorPlacement.EquallySpacedRectSide\",\"uuid\":\"d9face5b-155e-4e83-95c0-d581b737b6e3\"},{\"content\":{\"connectorIds\":[\"Out1\"],\"side\":\"RIGHT\"},\"type\":\"ConnectorPlacement.EquallySpacedRectSide\",\"uuid\":\"f965be1f-1639-4140-b9ea-f5e9efbe4150\"},{\"content\":{\"side\":\"TOP\"},\"type\":\"ConnectorPlacement.EquallySpacedRectSide\",\"uuid\":\"7c9c4b2b-011c-4482-afab-b6e67025a5e2\"}]},\"type\":\"ConnectorPlacement.EquallySpacedConnector\",\"uuid\":\"ec963004-117d-4f22-bb00-71f35201e6e2\"}],\"packageUris\":[\"http://schema.mathworks.com/mf0/Connector/R2020b\"],\"version\":\"1.0\"}"
  Bus Element Out1 : Outport  PortName=sPet
  Bus Element Out2 : Outport  Port=2  PortName=SUVR Volume
  Bus Element Out3 : Outport  Port=3  PortName=Surface Overlay
  wires:
  Bus Element In2/1 -> fs_align_pet/1(inVol)
  out_mri_nii/1(mri_nii) -> fs_register_pet/2(mri_nii)
  fs_align_pet/1(fsPetFile) -> fs_frame_mean/1(fsPetFile)
  in_pet_nii/2(vox2ras) -> cs_compute/2(vox2ras)
  in_pet_nii/1(PET) -> cs_compute/1(PET)
  fs_frame_mean/1(fsPet) -> fs_register_pet/1(fsPetFile)
  fs_register_pet/1(fsPet) -> in_pet_nii/1(PetFile)
  cs_compute/1(PetFile) -> tess_mri_mask/1(PetFile)

== system pet_integration_architecture/Freesurfer//Brainsuite/Freesurfer/LORIS Data Ingestor ==

== system pet_integration_architecture/Freesurfer//Brainsuite/Freesurfer/Linux ==
  Bus Element In1 : Inport  AllowServiceAccess=on  PortName=Client

== system pet_integration_architecture/Freesurfer//Brainsuite/Freesurfer/Windows ==
  Bus Element In1 : Inport  AllowServiceAccess=on  PortName=Client

== system pet_integration_architecture/Freesurfer//Brainsuite/Freesurfer/gitClone Brainstorm ==
  Bus Element In1 : Inport  AllowServiceAccess=on  PortName=sourceCode

== system pet_integration_architecture/Remote Data Server/Local WSL Store/bash Scripts ==

== system pet_integration_architecture/Remote Data Server/Local WSL Store/slurm Jobs ==

== system pet_integration_architecture/Remote Data Server/Local WSL Store/sshConnect ==

== system pet_integration_architecture/brainstorm SQLite Server/Freesurfer Processing Server/PETSurfer ==
  Bus Element Out1 : Outport  PortName=pet

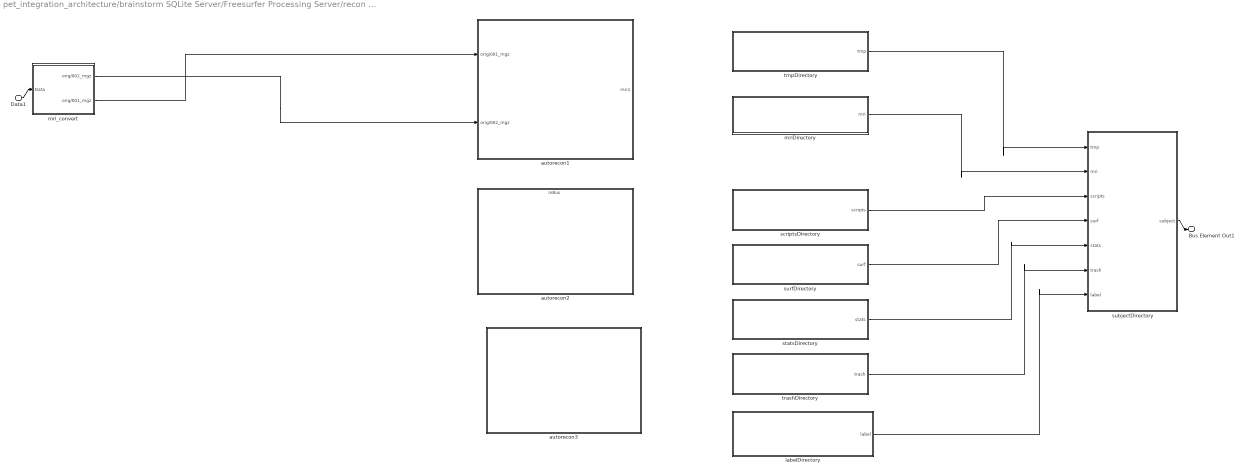
== system pet_integration_architecture/brainstorm SQLite Server/Freesurfer Processing Server/recon all ==
  Data1 : Inport  AllowServiceAccess=on  PortName=Data
  autorecon1 : Subsystem
      settings: PortSchema="{\"entries\":[{\"content\":{\"headerSize\":26,\"margin\":15,\"minimumSpacing\":25,\"sides\":[{\"content\":{\"connectorIds\":[\"In1\",\"In2\"]},\"type\":\"ConnectorPlacement.EquallySpacedRectSide\",\"uuid\":\"1ec5f43e-86ec-4420-9dd8-c30b843d5131\"},{\"content\":{\"connectorIds\":[\"Out1\"],\"side\":\"RIGHT\"},\"type\":\"ConnectorPlacement.EquallySpacedRectSide\",\"uuid\":\"372e8174-47dc-4989-909e-f78b7a521fdc\"},{\"content\":{\"side\":\"TOP\"},\"type\":\"ConnectorPlacement.EquallySpacedRectSide\",\"uuid\":\"cc67dfee-4023-44ab-9dd9-de9f078f7d77\"}]},\"type\":\"ConnectorPlacement.EquallySpacedConnector\",\"uuid\":\"fe3e41a6-8f67-44d2-abc6-74b481cf0464\"}],\"packageUris\":[\"http://schema.mathworks.com/mf0/Connector/R2020b\"],\"version\":\"1.0\"}"
  autorecon2 : Subsystem
      settings: PortSchema="{\"entries\":[{\"content\":{\"headerSize\":26,\"margin\":15,\"minimumSpacing\":25,\"sides\":[{\"content\":{},\"type\":\"ConnectorPlacement.EquallySpacedRectSide\",\"uuid\":\"d99db108-8c8a-4010-81b2-f142fbf318f5\"},{\"content\":{\"side\":\"RIGHT\"},\"type\":\"ConnectorPlacement.EquallySpacedRectSide\",\"uuid\":\"9190d96c-22e3-4cc9-a507-8f094dc67743\"},{\"content\":{\"connectorIds\":[\"In1\"],\"side\":\"TOP\"},\"type\":\"ConnectorPlacement.EquallySpacedRectSide\",\"uuid\":\"08b46875-eac1-4edb-b2eb-5598dd517a75\"}]},\"type\":\"ConnectorPlacement.EquallySpacedConnector\",\"uuid\":\"c8d2d02b-cf5a-431f-8876-22d36c8a9b33\"}],\"packageUris\":[\"http://schema.mathworks.com/mf0/Connector/R2020b\"],\"version\":\"1.0\"}"
  autorecon3 : Subsystem
      settings: PortSchema="{\"entries\":[{\"content\":{\"headerSize\":26,\"margin\":15,\"minimumSpacing\":25,\"sides\":[{\"content\":{},\"type\":\"ConnectorPlacement.EquallySpacedRectSide\",\"uuid\":\"d99db108-8c8a-4010-81b2-f142fbf318f5\"},{\"content\":{\"side\":\"RIGHT\"},\"type\":\"ConnectorPlacement.EquallySpacedRectSide\",\"uuid\":\"9190d96c-22e3-4cc9-a507-8f094dc67743\"},{\"content\":{\"side\":\"TOP\"},\"type\":\"ConnectorPlacement.EquallySpacedRectSide\",\"uuid\":\"08b46875-eac1-4edb-b2eb-5598dd517a75\"}]},\"type\":\"ConnectorPlacement.EquallySpacedConnector\",\"uuid\":\"c8d2d02b-cf5a-431f-8876-22d36c8a9b33\"}],\"packageUris\":[\"http://schema.mathworks.com/mf0/Connector/R2020b\"],\"version\":\"1.0\"}"
  labelDirectory : Subsystem
      settings: PortSchema="{\"entries\":[{\"content\":{\"headerSize\":26,\"margin\":15,\"minimumSpacing\":25,\"sides\":[{\"content\":{},\"type\":\"ConnectorPlacement.EquallySpacedRectSide\",\"uuid\":\"d99db108-8c8a-4010-81b2-f142fbf318f5\"},{\"content\":{\"connectorIds\":[\"Out1\"],\"side\":\"RIGHT\"},\"type\":\"ConnectorPlacement.EquallySpacedRectSide\",\"uuid\":\"9190d96c-22e3-4cc9-a507-8f094dc67743\"},{\"content\":{\"side\":\"TOP\"},\"type\":\"ConnectorPlacement.EquallySpacedRectSide\",\"uuid\":\"08b46875-eac1-4edb-b2eb-5598dd517a75\"}]},\"type\":\"ConnectorPlacement.EquallySpacedConnector\",\"uuid\":\"c8d2d02b-cf5a-431f-8876-22d36c8a9b33\"}],\"packageUris\":[\"http://schema.mathworks.com/mf0/Connector/R2020b\"],\"version\":\"1.0\"}"
  mriDirectory : Subsystem
      settings: PortSchema="{\"entries\":[{\"content\":{\"headerSize\":26,\"margin\":15,\"minimumSpacing\":25,\"sides\":[{\"content\":{},\"type\":\"ConnectorPlacement.EquallySpacedRectSide\",\"uuid\":\"d99db108-8c8a-4010-81b2-f142fbf318f5\"},{\"content\":{\"connectorIds\":[\"Out1\"],\"side\":\"RIGHT\"},\"type\":\"ConnectorPlacement.EquallySpacedRectSide\",\"uuid\":\"9190d96c-22e3-4cc9-a507-8f094dc67743\"},{\"content\":{\"side\":\"TOP\"},\"type\":\"ConnectorPlacement.EquallySpacedRectSide\",\"uuid\":\"08b46875-eac1-4edb-b2eb-5598dd517a75\"}]},\"type\":\"ConnectorPlacement.EquallySpacedConnector\",\"uuid\":\"c8d2d02b-cf5a-431f-8876-22d36c8a9b33\"}],\"packageUris\":[\"http://schema.mathworks.com/mf0/Connector/R2020b\"],\"version\":\"1.0\"}"
  mri_convert : Subsystem
      settings: PortSchema="{\"entries\":[{\"content\":{\"headerSize\":26,\"margin\":15,\"minimumSpacing\":25,\"sides\":[{\"content\":{\"connectorIds\":[\"In1\"]},\"type\":\"ConnectorPlacement.EquallySpacedRectSide\",\"uuid\":\"d99db108-8c8a-4010-81b2-f142fbf318f5\"},{\"content\":{\"connectorIds\":[\"Out1\",\"Out2\"],\"side\":\"RIGHT\"},\"type\":\"ConnectorPlacement.EquallySpacedRectSide\",\"uuid\":\"9190d96c-22e3-4cc9-a507-8f094dc67743\"},{\"content\":{\"side\":\"TOP\"},\"type\":\"ConnectorPlacement.EquallySpacedRectSide\",\"uuid\":\"08b46875-eac1-4edb-b2eb-5598dd517a75\"}]},\"type\":\"ConnectorPlacement.EquallySpacedConnector\",\"uuid\":\"c8d2d02b-cf5a-431f-8876-22d36c8a9b33\"}],\"packageUris\":[\"http://schema.mathworks.com/mf0/Connector/R2020b\"],\"version\":\"1.0\"}"
  scriptsDirectory : Subsystem
      settings: PortSchema="{\"entries\":[{\"content\":{\"headerSize\":26,\"margin\":15,\"minimumSpacing\":25,\"sides\":[{\"content\":{},\"type\":\"ConnectorPlacement.EquallySpacedRectSide\",\"uuid\":\"d99db108-8c8a-4010-81b2-f142fbf318f5\"},{\"content\":{\"connectorIds\":[\"Out1\"],\"side\":\"RIGHT\"},\"type\":\"ConnectorPlacement.EquallySpacedRectSide\",\"uuid\":\"9190d96c-22e3-4cc9-a507-8f094dc67743\"},{\"content\":{\"side\":\"TOP\"},\"type\":\"ConnectorPlacement.EquallySpacedRectSide\",\"uuid\":\"08b46875-eac1-4edb-b2eb-5598dd517a75\"}]},\"type\":\"ConnectorPlacement.EquallySpacedConnector\",\"uuid\":\"c8d2d02b-cf5a-431f-8876-22d36c8a9b33\"}],\"packageUris\":[\"http://schema.mathworks.com/mf0/Connector/R2020b\"],\"version\":\"1.0\"}"
  statsDirectory : Subsystem
      settings: PortSchema="{\"entries\":[{\"content\":{\"headerSize\":26,\"margin\":15,\"minimumSpacing\":25,\"sides\":[{\"content\":{},\"type\":\"ConnectorPlacement.EquallySpacedRectSide\",\"uuid\":\"d99db108-8c8a-4010-81b2-f142fbf318f5\"},{\"content\":{\"connectorIds\":[\"Out1\"],\"side\":\"RIGHT\"},\"type\":\"ConnectorPlacement.EquallySpacedRectSide\",\"uuid\":\"9190d96c-22e3-4cc9-a507-8f094dc67743\"},{\"content\":{\"side\":\"TOP\"},\"type\":\"ConnectorPlacement.EquallySpacedRectSide\",\"uuid\":\"08b46875-eac1-4edb-b2eb-5598dd517a75\"}]},\"type\":\"ConnectorPlacement.EquallySpacedConnector\",\"uuid\":\"c8d2d02b-cf5a-431f-8876-22d36c8a9b33\"}],\"packageUris\":[\"http://schema.mathworks.com/mf0/Connector/R2020b\"],\"version\":\"1.0\"}"
  subjectDirectory : Subsystem
      settings: PortSchema="{\"entries\":[{\"content\":{\"headerSize\":26,\"margin\":15,\"minimumSpacing\":25,\"sides\":[{\"content\":{\"connectorIds\":[\"In1\",\"In2\",\"In3\",\"In4\",\"In5\",\"In6\",\"In7\"]},\"type\":\"ConnectorPlacement.EquallySpacedRectSide\",\"uuid\":\"d99db108-8c8a-4010-81b2-f142fbf318f5\"},{\"content\":{\"connectorIds\":[\"Out1\"],\"side\":\"RIGHT\"},\"type\":\"ConnectorPlacement.EquallySpacedRectSide\",\"uuid\":\"9190d96c-22e3-4cc9-a507-8f094dc67743\"},{\"content\":{\"side\":\"TOP\"},\"type\":\"ConnectorPlacement.EquallySpacedRectSide\",\"uuid\":\"08b46875-eac1-4edb-b2eb-5598dd517a75\"}]},\"type\":\"ConnectorPlacement.EquallySpacedConnector\",\"uuid\":\"c8d2d02b-cf5a-431f-8876-22d36c8a9b33\"}],\"packageUris\":[\"http://schema.mathworks.com/mf0/Connector/R2020b\"],\"version\":\"1.0\"}"
  surfDirectory : Subsystem
      settings: PortSchema="{\"entries\":[{\"content\":{\"headerSize\":26,\"margin\":15,\"minimumSpacing\":25,\"sides\":[{\"content\":{},\"type\":\"ConnectorPlacement.EquallySpacedRectSide\",\"uuid\":\"d99db108-8c8a-4010-81b2-f142fbf318f5\"},{\"content\":{\"connectorIds\":[\"Out1\"],\"side\":\"RIGHT\"},\"type\":\"ConnectorPlacement.EquallySpacedRectSide\",\"uuid\":\"9190d96c-22e3-4cc9-a507-8f094dc67743\"},{\"content\":{\"side\":\"TOP\"},\"type\":\"ConnectorPlacement.EquallySpacedRectSide\",\"uuid\":\"08b46875-eac1-4edb-b2eb-5598dd517a75\"}]},\"type\":\"ConnectorPlacement.EquallySpacedConnector\",\"uuid\":\"c8d2d02b-cf5a-431f-8876-22d36c8a9b33\"}],\"packageUris\":[\"http://schema.mathworks.com/mf0/Connector/R2020b\"],\"version\":\"1.0\"}"
  tmpDirectory : Subsystem
      settings: PortSchema="{\"entries\":[{\"content\":{\"headerSize\":26,\"margin\":15,\"minimumSpacing\":25,\"sides\":[{\"content\":{},\"type\":\"ConnectorPlacement.EquallySpacedRectSide\",\"uuid\":\"d99db108-8c8a-4010-81b2-f142fbf318f5\"},{\"content\":{\"connectorIds\":[\"Out1\"],\"side\":\"RIGHT\"},\"type\":\"ConnectorPlacement.EquallySpacedRectSide\",\"uuid\":\"9190d96c-22e3-4cc9-a507-8f094dc67743\"},{\"content\":{\"side\":\"TOP\"},\"type\":\"ConnectorPlacement.EquallySpacedRectSide\",\"uuid\":\"08b46875-eac1-4edb-b2eb-5598dd517a75\"}]},\"type\":\"ConnectorPlacement.EquallySpacedConnector\",\"uuid\":\"c8d2d02b-cf5a-431f-8876-22d36c8a9b33\"}],\"packageUris\":[\"http://schema.mathworks.com/mf0/Connector/R2020b\"],\"version\":\"1.0\"}"
  trashDirectory : Subsystem
      settings: PortSchema="{\"entries\":[{\"content\":{\"headerSize\":26,\"margin\":15,\"minimumSpacing\":25,\"sides\":[{\"content\":{},\"type\":\"ConnectorPlacement.EquallySpacedRectSide\",\"uuid\":\"d99db108-8c8a-4010-81b2-f142fbf318f5\"},{\"content\":{\"connectorIds\":[\"Out1\"],\"side\":\"RIGHT\"},\"type\":\"ConnectorPlacement.EquallySpacedRectSide\",\"uuid\":\"9190d96c-22e3-4cc9-a507-8f094dc67743\"},{\"content\":{\"side\":\"TOP\"},\"type\":\"ConnectorPlacement.EquallySpacedRectSide\",\"uuid\":\"08b46875-eac1-4edb-b2eb-5598dd517a75\"}]},\"type\":\"ConnectorPlacement.EquallySpacedConnector\",\"uuid\":\"c8d2d02b-cf5a-431f-8876-22d36c8a9b33\"}],\"packageUris\":[\"http://schema.mathworks.com/mf0/Connector/R2020b\"],\"version\":\"1.0\"}"
  Bus Element Out1 : Outport  PortName=subject
  wires:
  Data1/1 -> mri_convert/1(Data)
  labelDirectory/1(label) -> subjectDirectory/7(label)
  scriptsDirectory/1(scripts) -> subjectDirectory/3(scripts)
  mriDirectory/1(mri) -> subjectDirectory/2(mri)
  trashDirectory/1(trash) -> subjectDirectory/6(trash)
  statsDirectory/1(stats) -> subjectDirectory/5(stats)
  surfDirectory/1(surf) -> subjectDirectory/4(surf)
  tmpDirectory/1(tmp) -> subjectDirectory/1(tmp)
  mri_convert/1(orig/002_mgz) -> autorecon1/2(orig/002_mgz)
  mri_convert/2(orig/001_mgz) -> autorecon1/1(orig/001_mgz)
  subjectDirectory/1(subject) -> Bus Element Out1/1

== system pet_integration_architecture/brainstorm SQLite Server/Remote Data Server/ sourceData ==
  Bus Element Out1 : Outport  AllowServiceAccess=on  PortName=remote

== system pet_integration_architecture/brainstorm SQLite Server/Remote Data Server/Home ==
  Bus Element Out1 : Outport  AllowServiceAccess=on  PortName=sourceCode

== system pet_integration_architecture/brainstorm SQLite Server/Remote Data Server/derivativesData ==

== system pet_integration_architecture/brainstorm database/Brainstorm data server/channel_ ==
  Bus Element In1 : Inport  PortName=FileName

== system pet_integration_architecture/brainstorm database/Brainstorm data server/channel_1 ==
  Bus Element In1 : Inport  PortName=FileName

== system pet_integration_architecture/brainstorm database/Brainstorm data server/data_ ==
  Bus Element In1 : Inport  PortName=FileName

== system pet_integration_architecture/brainstorm database/Brainstorm data server/pet_ ==
  Bus Element In1 : Inport  PortName=FileName
  Bus Element In2 : Inport  Port=2  PortName=Tracer
  Bus Element In3 : Inport  Port=3  PortName=nFrames

== system pet_integration_architecture/brainstorm database/Brainstorm data server/subjectimage_ ==
  Bus Element In1 : Inport  PortName=FileName

== system pet_integration_architecture/brainstorm database/Brainstorm data server/tess_ ==
  Bus Element In2 : Inport  PortName=FileName

== system pet_integration_architecture/brainstorm database/Brainstorm metadata /AnatomyFile ==
  Bus Element In1 : Inport  PortName=Subject
  Bus Element Out1 : Outport  PortName=FileName
  Bus Element Out2 : Outport  Port=2  PortName=SubType

== system pet_integration_architecture/brainstorm database/Brainstorm metadata /FunctionalFile ==
  Bus Element In1 : Inport  PortName=Study
  Bus Element Out1 : Outport  PortName=FileName

== system pet_integration_architecture/brainstorm database/Brainstorm metadata /PetFile ==
  Bus Element In2 : Inport  PortName=Study
  Bus Element In1 : Inport  Port=2  PortName=Subject
  Bus Element Out1 : Outport  PortName=FileName
  Bus Element Out2 : Outport  Port=2  PortName=Tracer
  Bus Element Out3 : Outport  Port=3  PortName=nFrames

== system pet_integration_architecture/brainstorm database/Brainstorm metadata /Protocol ==
  note: db_template( 'ProtocolStudies' )
  note: db_template( 'ProtocolSubjects' )
  note: db_template( 'ProtocolInfo' )
  ProtocolInfo : Subsystem
      settings: PortSchema="{\"entries\":[{\"content\":{\"headerSize\":26,\"margin\":15,\"minimumSpacing\":25,\"sides\":[{\"content\":{},\"type\":\"ConnectorPlacement.EquallySpacedRectSide\",\"uuid\":\"e452b68a-48a0-46a4-9e6b-6a7ab63d76ba\"},{\"content\":{\"side\":\"RIGHT\"},\"type\":\"ConnectorPlacement.EquallySpacedRectSide\",\"uuid\":\"bfc23a96-7562-4108-a377-c6d682106293\"},{\"content\":{\"side\":\"TOP\"},\"type\":\"ConnectorPlacement.EquallySpacedRectSide\",\"uuid\":\"898805eb-9365-4e37-9830-3cdbb7191da7\"}]},\"type\":\"ConnectorPlacement.EquallySpacedConnector\",\"uuid\":\"9a83eb3e-c81f-4df4-a7ca-e8a116b52f55\"}],\"packageUris\":[\"http://schema.mathworks.com/mf0/Connector/R2020b\"],\"version\":\"1.0\"}"
  ProtocolStudies : Subsystem
      settings: PortSchema="{\"entries\":[{\"content\":{\"headerSize\":26,\"margin\":15,\"minimumSpacing\":25,\"sides\":[{\"content\":{},\"type\":\"ConnectorPlacement.EquallySpacedRectSide\",\"uuid\":\"e452b68a-48a0-46a4-9e6b-6a7ab63d76ba\"},{\"content\":{\"side\":\"RIGHT\"},\"type\":\"ConnectorPlacement.EquallySpacedRectSide\",\"uuid\":\"bfc23a96-7562-4108-a377-c6d682106293\"},{\"content\":{\"side\":\"TOP\"},\"type\":\"ConnectorPlacement.EquallySpacedRectSide\",\"uuid\":\"898805eb-9365-4e37-9830-3cdbb7191da7\"}]},\"type\":\"ConnectorPlacement.EquallySpacedConnector\",\"uuid\":\"9a83eb3e-c81f-4df4-a7ca-e8a116b52f55\"}],\"packageUris\":[\"http://schema.mathworks.com/mf0/Connector/R2020b\"],\"version\":\"1.0\"}"
  ProtocolSubjects : Subsystem
      settings: PortSchema="{\"entries\":[{\"content\":{\"headerSize\":26,\"margin\":15,\"minimumSpacing\":25,\"sides\":[{\"content\":{},\"type\":\"ConnectorPlacement.EquallySpacedRectSide\",\"uuid\":\"e452b68a-48a0-46a4-9e6b-6a7ab63d76ba\"},{\"content\":{\"side\":\"RIGHT\"},\"type\":\"ConnectorPlacement.EquallySpacedRectSide\",\"uuid\":\"bfc23a96-7562-4108-a377-c6d682106293\"},{\"content\":{\"side\":\"TOP\"},\"type\":\"ConnectorPlacement.EquallySpacedRectSide\",\"uuid\":\"898805eb-9365-4e37-9830-3cdbb7191da7\"}]},\"type\":\"ConnectorPlacement.EquallySpacedConnector\",\"uuid\":\"9a83eb3e-c81f-4df4-a7ca-e8a116b52f55\"}],\"packageUris\":[\"http://schema.mathworks.com/mf0/Connector/R2020b\"],\"version\":\"1.0\"}"
  Bus Element Out1 : Outport  PortName=Id

== system pet_integration_architecture/brainstorm database/Brainstorm metadata /Study ==
  note: db_template( 'ProtocolStudies' )
  Bus Element In2 : Inport  PortName=Protocol
  Bus Element In1 : Inport  Port=2  PortName=Subject
  Bus Element Out1 : Outport  PortName=Id

== system pet_integration_architecture/brainstorm database/Brainstorm metadata /Subject ==
  note: db_template( 'ProtocolSubjects' )
  Bus Element In1 : Inport  PortName=Protocol
  Bus Element Out2 : Outport  PortName=Id

== system pet_integration_architecture/brainstorm io/import_pet/VolType ==
  Bus Element Out1 : Outport  PortName=volType
